simulink library "aeroSurface_ul"  (R2018b)
settings: Solver=VariableStepAuto  StartTime=0.0  StopTime=10.0  RelTol=1e-3
values from neighbouring files (symbols this model uses):
  RBody2Surf = [xUnitVec(:)';      yUnitVec(:)';      zUnitvec(:)']    [aeroSurface_init.m]
  RSurf2Body = inv(RBody2Surf)    [aeroSurface_init.m]
libraries: vrlib x3
settings Model: Creator=mcobb  LastModifiedBy=mcobb

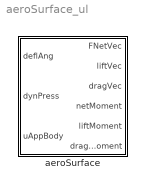
== system aeroSurface_ul ==
  aeroSurface : Subsystem  mask{rAeroCent=[1 0 0], uSpan=[0 1 0], uChord=[0 0 1], ARef=1, ClFitParams=[1 0], CdFitParams=[1 0 1]}
      mask prompts: rAeroCent "Aerodynamic center position vector"; uSpan "Spanwise positive rotation unit vector"; uChord "Increasing chord direction in body frame unit vector"; ARef "Reference area"; ClFitParams "Lift coefficient fit parameters"; CdFitParams "Drag coefficient fit parameters"
      mask help:
      | Block to model a generic planar aerodynamic surface that rotates about its span.
      |
      | Note that all vectors are in the body fixed coordinate system and are relative to the origin of that coordinate system (which is probably the center of mass).
      |
      | Click the help button for more details on the spanwise positive rotation vector.
      |
      | 5/14/19
      | -MC
      mask init:
      | aeroSurface_init
      mask Help: One of the inputs to this block is the spanwise positive rotation vector.  This is the vector that define exactly what constitutes a positive or negative deflection of the control surface.  If the signal into the deflAng is positive, it is interpreted to mean that this planar surface is rotated by that amount about this unit vector.
      mask DialogControl Container3 Prompt: Geometric Parameters
      mask DialogControl Container4 Prompt: Aerodynamic Parameters

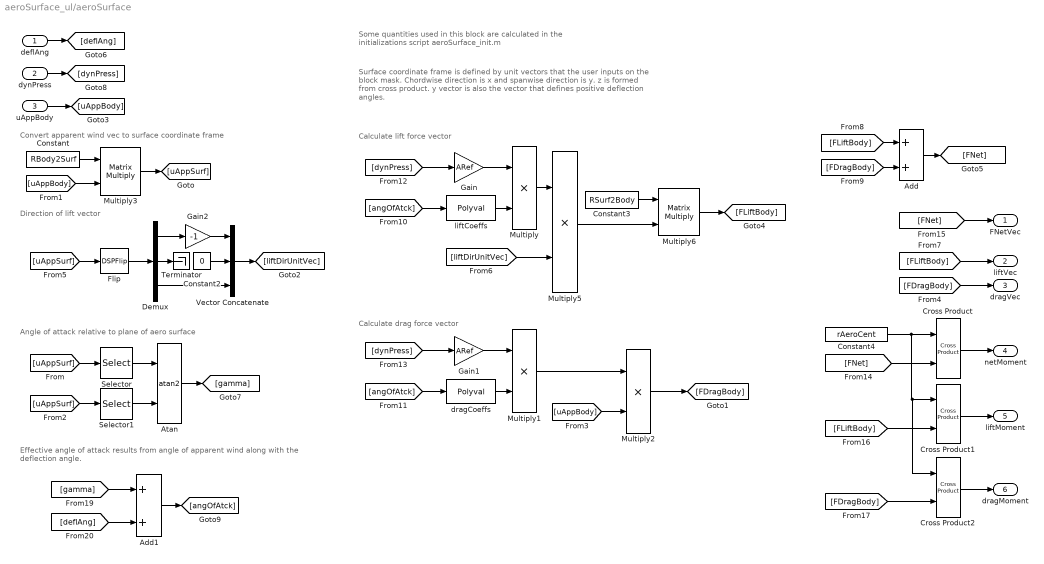
== system aeroSurface_ul/aeroSurface ==
  note: Effective angle of attack results from angle of apparent
      | wind along with the deflection angle.
  note: Calculate drag force vector
  note: Calculate lift force vector
  note: Surface coordinate frame is defined by unit vectors that the
      | user inputs on the block mask. Chordwise direction is x and
      | spanwise direction is y. z is formed from cross product. y
      | vector is also the vector that defines positive deflection angles.
  note: Convert apparent wind vec to surface coordinate frame
  note: Direction of lift vector
  note: Angle of attack relative to plane of aero surface
  note: Some quantities used in this block are calculated
      | in the initializations script aeroSurface_init.m
  deflAng : Inport
  dynPress : Inport  Port=2
  uAppBody : Inport  Port=3
  Add : Sum
  Add1 : Sum
  Atan : Trigonometry  Operator=atan2
  Constant : Constant  Value=RBody2Surf
  Constant2 : Constant  Value=0
  Constant3 : Constant  Value=RSurf2Body
  Constant4 : Constant  Value=rAeroCent
  Cross Product : vrlib/Utilities/Cross Product
      settings: SourceProductBaseCode=VR
  Cross Product1 : vrlib/Utilities/Cross Product
      settings: SourceProductBaseCode=VR
  Cross Product2 : vrlib/Utilities/Cross Product
      settings: SourceProductBaseCode=VR
  Demux : Demux  Outputs=3
  Flip : DSPFlip
  Gain : Gain  Gain=ARef
  Gain1 : Gain  Gain=ARef
  Gain2 : Gain  Gain=-1
  Multiply{,1..2,5} (4 alike) : Product
  Multiply3 : Product  Multiplication=Matrix(*)
  Multiply6 : Product  Multiplication=Matrix(*)
  Selector : Selector  InputPortWidth=3  IndexOptions=Index vector (dialog)  Indices=3  OutputSizes=1
  Selector1 : Selector  InputPortWidth=3  IndexOptions=Index vector (dialog)  Indices=1  OutputSizes=1
  Terminator : Terminator
  Vector Concatenate : Concatenate  NumInputs=3
  dragCoeffs : Polyval  Coefs=CdFitParams
  liftCoeffs : Polyval  Coefs=ClFitParams
  FNetVec : Outport
  liftVec : Outport  Port=2
  dragVec : Outport  Port=3
  netMoment : Outport  Port=4
  liftMoment : Outport  Port=5
  dragMoment : Outport  Port=6
  wires:
  Add1/1 -> [angOfAtck]
  [deflAng] -> Add1/2
  [gamma] -> Add1/1
  deflAng/1 -> [deflAng]
  Flip/1 -> Demux/1
  [FDragBody] -> Cross Product2/2
  [FLiftBody] -> Cross Product1/2
  Cross Product2/1 -> dragMoment/1
  Constant4/1 -> Cross Product/1, Cross Product1/1, Cross Product2/1
  Cross Product1/1 -> liftMoment/1
  [FNet] -> Cross Product/2
  Cross Product/1 -> netMoment/1
  [FNet] -> FNetVec/1
  [FDragBody] -> Add/2
  [FLiftBody] -> Add/1
  Add/1 -> [FNet]
  [FLiftBody] -> liftVec/1
  Multiply6/1 -> [FLiftBody]
  Constant3/1 -> Multiply6/1
  Multiply5/1 -> Multiply6/2
  Multiply/1 -> Multiply5/1
  [liftDirUnitVec] -> Multiply5/2
  Vector Concatenate/1 -> [liftDirUnitVec]
  Demux/3 -> Vector Concatenate/3
  Constant2/1 -> Vector Concatenate/2
  Demux/1 -> Gain2/1
  Demux/2 -> Terminator/1
  [uAppSurf] -> Flip/1
  [FDragBody] -> dragVec/1
  Multiply2/1 -> [FDragBody]
  [uAppSurf] -> Selector1/1
  [uAppSurf] -> Selector/1
  Multiply3/1 -> [uAppSurf]
  Constant/1 -> Multiply3/1
  [uAppBody] -> Multiply3/2
  Multiply1/1 -> Multiply2/1
  [uAppBody] -> Multiply2/2
  dragCoeffs/1 -> Multiply1/2
  [dynPress] -> Gain1/1
  Gain1/1 -> Multiply1/1
  Gain/1 -> Multiply/1
  liftCoeffs/1 -> Multiply/2
  [dynPress] -> Gain/1
  [angOfAtck] -> dragCoeffs/1
  [angOfAtck] -> liftCoeffs/1
  Atan/1 -> [gamma]
  Selector1/1 -> Atan/2
  Selector/1 -> Atan/1
  uAppBody/1 -> [uAppBody]
  dynPress/1 -> [dynPress]
  Gain2/1 -> Vector Concatenate/1
